simulink model "Simulink_ZT_P1P2"  (R2021a)
settings: Solver=VariableStepAuto  StartTime=0.0  StopTime=10.0  RelTol=1e-3
values from neighbouring files (symbols this model uses):
  u0 = 0    [Praktikum.m]    (also in Praktikum_1.m = 0.2)
  x0 = [0 0 0 0]    [Praktikum.m]    (also in Praktikum_1.m = [5 0 0 0])
  ZRM = ZRMGummi    [Praktikum.m]    (also in Praktikum_1.m; calcZRM.m = ss(A,bv,cT,d))
settings Model: Creator=janis  LastModifiedBy=janis

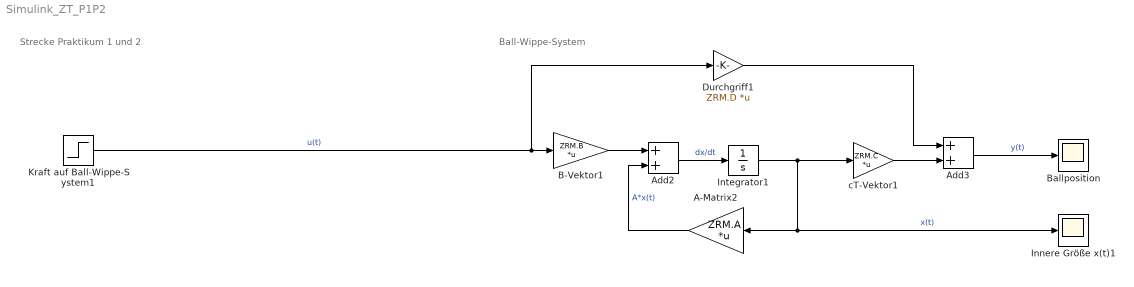
== system Simulink_ZT_P1P2 ==
  note: Strecke Praktikum 1 und 2
  note: Ball-Wippe-System
  A-Matrix2 : Gain  Gain=ZRM.A  Multiplication=Matrix(K*u) (u vector)
  Add2 : Sum
  Add3 : Sum
  B-Vektor1 : Gain  Gain=ZRM.B  Multiplication=Matrix(K*u) (u vector)
  Ballposition : Scope
  Durchgriff1 : Gain  Gain=ZRM.D  Multiplication=Matrix(K*u)
  Innere Größe x(t)1 : Scope
  Integrator1 : Integrator  InitialCondition=x0
  Kraft auf Ball-Wippe-System1 : Step  After=u0  SampleTime=0
  cT-Vektor1 : Gain  Gain=ZRM.C  Multiplication=Matrix(K*u) (u vector)
  wires:
  B-Vektor1/1 -> Add2/1
  A-Matrix2/1 -> Add2/2  "A*x(t)"
  Integrator1/1 -> Innere Größe x(t)1/1, A-Matrix2/1, cT-Vektor1/1  "x(t)"
  Add2/1 -> Integrator1/1  "dx/dt"
  cT-Vektor1/1 -> Add3/2
  Kraft auf Ball-Wippe-System1/1 -> Durchgriff1/1, B-Vektor1/1  "u(t)"
  Add3/1 -> Ballposition/1  "y(t)"
  Durchgriff1/1 -> Add3/1
